simulink library "VariousLibrary"  (R2016b)
settings: Solver=VariableStepAuto  StartTime=0.0  StopTime=10.0  RelTol=1e-3
values from neighbouring files (symbols this model uses):
  currentMaximum = 35.0    [ModelDictionary.sldd]
  currentNominal = 15.0    [ModelDictionary.sldd]
  currentTimeMaximum = 40.0    [ModelDictionary.sldd]
undefined symbols (not defined in the file or in its folder): Joints
settings Model: Creator=Nathan  LastModifiedBy=march

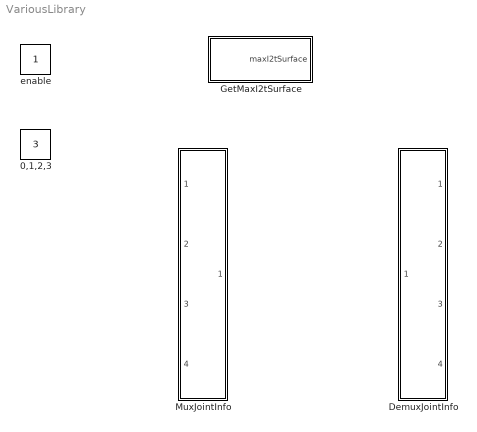
== system VariousLibrary ==
  0,1,2,3 : Constant  Value=3
      settings: OpenFcn=|
      | b = get_param(gcb,'value');
      | if (strcmp(b,'1')),
      |   set_param (gcb,'value','2');
      | elseif (strcmp(b,'2')),
      |  set_param (gcb,'value','3');
      | elseif (strcmp(b,'3')),
      |  set_param (gcb,'value','1');
      | end;
  DemuxJointInfo : Subsystem
  GetMaxI2tSurface : Subsystem
  MuxJointInfo : Subsystem
  enable : Constant
      settings: OpenFcn=|
      | b = get_param(gcb,'value');
      | if (strcmp(b,'1')),
      |   set_param (gcb,'value','0');
      | else
      |   set_param(gcb,'value','1');
      | end;

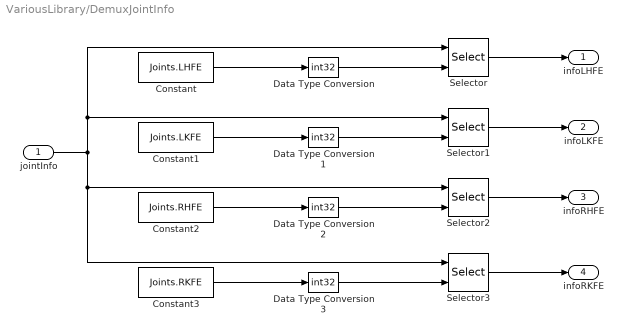
== system VariousLibrary/DemuxJointInfo ==
  jointInfo : Inport
  Constant : Constant  Value=Joints.LHFE
  Constant1 : Constant  Value=Joints.LKFE
  Constant2 : Constant  Value=Joints.RHFE
  Constant3 : Constant  Value=Joints.RKFE
  Data Type Conversion{,1..3} (4 alike) : DataTypeConversion  OutDataTypeStr=int32  RndMeth=Nearest
  Selector{,1..3} (4 alike) : Selector  InputPortWidth=4  IndexOptions=Index vector (port)  Indices=[1 3]  OutputSizes=1
  infoLHFE : Outport
  infoLKFE : Outport  Port=2
  infoRHFE : Outport  Port=3
  infoRKFE : Outport  Port=4
  wires:
  Data Type Conversion3/1 -> Selector3/2
  Data Type Conversion2/1 -> Selector2/2
  Data Type Conversion1/1 -> Selector1/2
  Data Type Conversion/1 -> Selector/2
  Selector/1 -> infoLHFE/1
  Selector1/1 -> infoLKFE/1
  Selector2/1 -> infoRHFE/1
  Selector3/1 -> infoRKFE/1
  jointInfo/1 -> Selector/1, Selector1/1, Selector3/1, Selector2/1
  Constant/1 -> Data Type Conversion/1
  Constant1/1 -> Data Type Conversion1/1
  Constant2/1 -> Data Type Conversion2/1
  Constant3/1 -> Data Type Conversion3/1

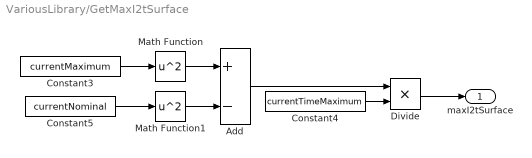
== system VariousLibrary/GetMaxI2tSurface ==
  Add : Sum  Inputs=+-
  Constant3 : Constant  Value=currentMaximum  VectorParams1D=off  SampleTime=-1
  Constant4 : Constant  Value=currentTimeMaximum  VectorParams1D=off  SampleTime=-1
  Constant5 : Constant  Value=currentNominal  VectorParams1D=off  SampleTime=-1
  Divide : Product  Inputs=**
  Math Function : Math  Operator=square  SaturateOnIntegerOverflow=on
  Math Function1 : Math  Operator=square  SaturateOnIntegerOverflow=on
  maxI2tSurface : Outport
  wires:
  Divide/1 -> maxI2tSurface/1
  Constant3/1 -> Math Function/1
  Constant5/1 -> Math Function1/1
  Math Function/1 -> Add/1
  Math Function1/1 -> Add/2
  Add/1 -> Divide/1
  Constant4/1 -> Divide/2

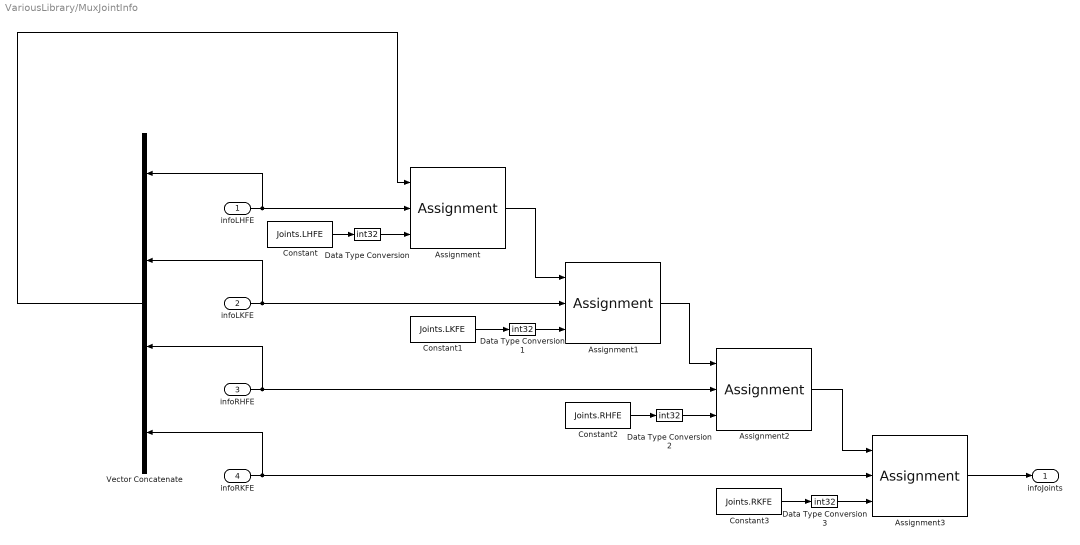
== system VariousLibrary/MuxJointInfo ==
  infoLHFE : Inport
  infoLKFE : Inport  Port=2
  infoRHFE : Inport  Port=3
  infoRKFE : Inport  Port=4
  Assignment{,1..3} (4 alike) : Assignment  DiagnosticForDimensions=Warning  IndexOptions=Index vector (port)  Indices=1  OutputSizes=1
  Constant : Constant  Value=Joints.LHFE
  Constant1 : Constant  Value=Joints.LKFE
  Constant2 : Constant  Value=Joints.RHFE
  Constant3 : Constant  Value=Joints.RKFE
  Data Type Conversion{,1..3} (4 alike) : DataTypeConversion  OutDataTypeStr=int32  RndMeth=Nearest
  Vector Concatenate : Concatenate  NumInputs=4  ConcatenateDimension=2
  infoJoints : Outport
  wires:
  Data Type Conversion3/1 -> Assignment3/3
  Data Type Conversion2/1 -> Assignment2/3
  Data Type Conversion1/1 -> Assignment1/3
  Data Type Conversion/1 -> Assignment/3
  infoLKFE/1 -> Assignment1/2, Vector Concatenate/2
  infoRKFE/1 -> Assignment3/2, Vector Concatenate/4
  infoRHFE/1 -> Assignment2/2, Vector Concatenate/3
  infoLHFE/1 -> Vector Concatenate/1, Assignment/2
  Vector Concatenate/1 -> Assignment/1
  Constant/1 -> Data Type Conversion/1
  Assignment/1 -> Assignment1/1
  Constant1/1 -> Data Type Conversion1/1
  Assignment1/1 -> Assignment2/1
  Constant2/1 -> Data Type Conversion2/1
  Assignment2/1 -> Assignment3/1
  Constant3/1 -> Data Type Conversion3/1
  Assignment3/1 -> infoJoints/1
